simulink model "PWMDBTest"  (R2016b)
settings: Solver=ode5  StartTime=0.0  StopTime=inf  FixedStep=0.001  RelTol=1e-3  EnableMultiTasking=on
libraries: dcpctrl x3
settings Model: SimulationMode=external  Creator=julianleland  LastModifiedBy=julianleland
settings OptimizationCC: LifeSpan=inf
settings DebuggingCC: SFUnexpectedBacktrackingDiag=warning  SFNoUnconditionalDefaultTransitionDiag=warning  SFExecutionAtInitializationDiag=none
settings HardwareCC: ProdBitPerLong=64  ProdHWDeviceType=Intel->x86-64 (Mac OS X)  TargetBitPerLong=64  TargetBitPerPointer=64  TargetIntDivRoundTo=Zero  TargetEndianess=LittleEndian  TargetWordSize=64  TargetHWDeviceType=Intel->x86-64
settings RTWCC: SystemTargetFile=sldrt.tlc  TemplateMakefile=sldrt.tmf  Description=Simulink Desktop Real-Time  RTWCompilerOptimization=on
settings CodeAppCC: MaxIdLength=95
settings SimulinkDesktopRealTimeCC: TargetPreCompLibLocation=/Applications/MATLAB_R2016b.app/toolbox/sldrt/lib/maci64  TargetLangStandard=C89/C90 (ANSI)  SupportVariableSizeSignals=off
settings ConfigComp: CovMetricSettings=dw  CovHtmlReporting=on  CovSaveCumulativeToWorkspaceVar=on  CovSaveSingleToWorkspaceVar=on  CovExternalEMLEnable=off

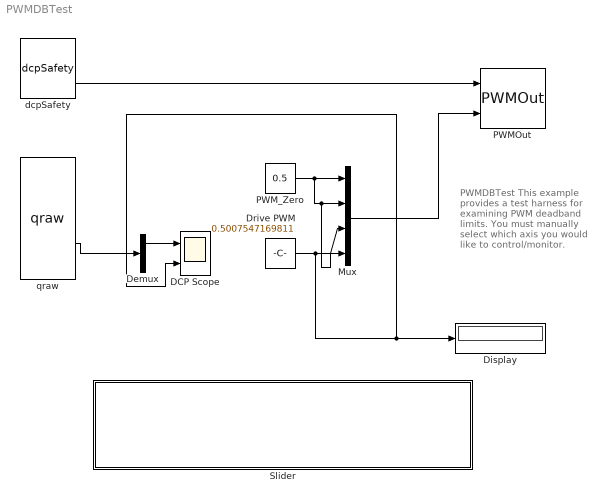
== system PWMDBTest ==
  note: PWMDBTest
      |
      | This example provides a test harness for examining PWM deadband limits. You must manually select which axis you would like to control/monitor.
  DCP Scope : Scope  NumInputPorts=2
  Demux : Demux  Outputs=2
  Display : Display
  Drive PWM : Constant  Value=0.5007547169811
  Mux : Mux
  PWMOut : dcpctrl/PWMOut
  PWM_Zero : Constant  Value=0.5
  Slider : Subsystem  DialogController=hmiCreateDDGDialog  IsWebBlock=on  mask(MWDashboardBlock){webBlockId=95684291-3303-4c9b-ad11-345a57b29d60, webBlockType=slider, ShowInLibBrowser=on, ShowInitialText=on, HMISrcModelName=PWMDBTest}
      mask prompts: webBlockId "WebBlock Id"; webBlockType "WebBlock Type"; HMISrcModelName "Source Model"
      mask help: SimulinkHMI:dialogs:SliderDialogDesc
      mask Help: helpview([docroot '/mapfiles/simulink.map'], 'hmi_slider')
      mask Display:
      | if strcmp(get_param(bdroot(gcb),'BlockDiagramType'), 'library')
      |     image([(matlabroot) '/toolbox/simulink/hmi/icons/Slider.png']);
      | end
  dcpSafety : dcpctrl/dcpSafety
  qraw : dcpctrl/qraw
  wires:
  dcpSafety/2 -> PWMOut/1
  Mux/1 -> PWMOut/2
  PWM_Zero/1 -> Mux/4, Mux/2, Mux/1
  qraw/4 -> Demux/1
  Drive PWM/1 -> Mux/3, DCP Scope/2, Display/1
  Demux/1 -> DCP Scope/1

== system PWMDBTest/Slider ==
